simulink model "CCI"  (R2015a)
settings: Solver=ode45  StartTime=0.0  StopTime=Inf  RelTol=1e-3
libraries: commfilt2 x6, commdigbbndam3 x3, commrandsrc2 x2, commchan3 x1, commsink2 x1
settings Model: Creator=konstantis  LastModifiedBy=arlim

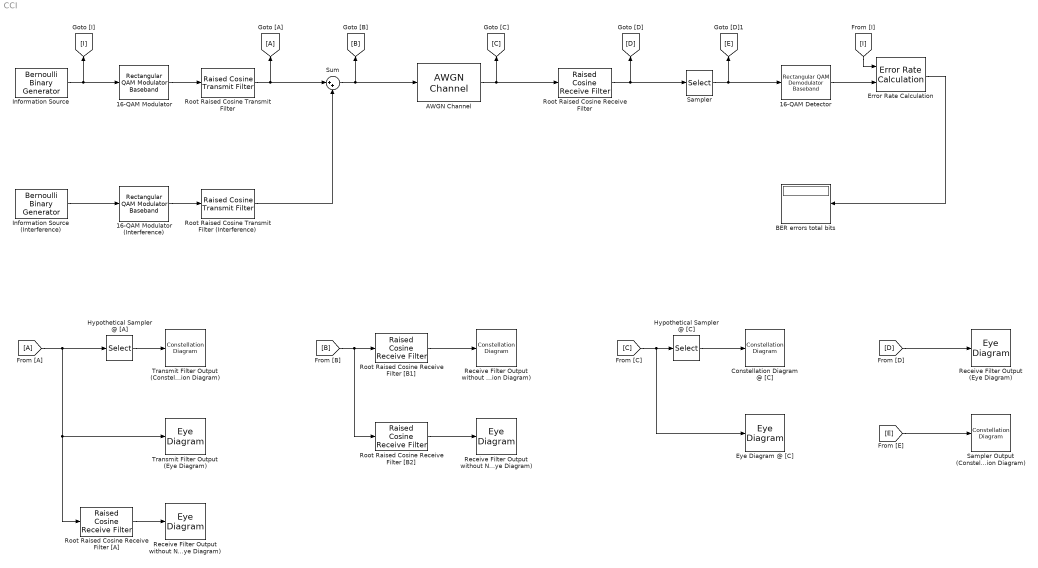
== system CCI ==
  16-QAM Detector : commdigbbndam3/Rectangular QAM Demodulator Baseband  M=16  PowType=Average Power  MinDist=2  AvgPow=1  PeakPow=1  Ph=0  Dec=Gray  Mapping=[0:15]  OutType=Bit  DecType=Hard decision  VarSource=Dialog  Variance=1  outDtype1=Inherit via internal rule  outDtype2=Inherit via internal rule  derotateFactorWordLen=16  denormFactorWordLen=16  prodOutWordLen=32  prodOutRoundingMode=Floor  prodOutOverflowMode=Wrap  sumWordLen=32
  16-QAM Modulator : commdigbbndam3/Rectangular QAM Modulator Baseband  M=16  InType=Bit  Enc=Gray  Mapping=[0:15]  PowType=Average Power  MinDist=2  AvgPow=1  PeakPow=1  Ph=0  outDtype=double  outWordLen=16  outUDDataType=sfix(16)  outFracLenMode=Best precision  outFracLen=15
  16-QAM Modulator (Interference) : commdigbbndam3/Rectangular QAM Modulator Baseband  M=16  InType=Bit  Enc=Gray  Mapping=[0:15]  PowType=Average Power  MinDist=2  AvgPow=.01  PeakPow=1  Ph=0  outDtype=double  outWordLen=16  outUDDataType=sfix(16)  outFracLenMode=Best precision  outFracLen=15
  AWGN Channel : commchan3/AWGN Channel  InputProcessing=Columns as channels (frame based)  seed=67  noiseMode="Signal to noise ratio  (SNR)"  EbNodB=10  EsNodB=10  SNRdB=15  bitsPerSym=1  Ps=1.01  Tsym=1  variance=1
  BER errors total bits : Display
      settings: Format=short_e
  Constellation Diagram @ [C] : ConstellationDiagram
  Error Rate Calculation : commsink2/Error Rate Calculation  N=128  st_delay=0  cp_mode=Entire frame  subframe=[64:10000]  PMode=Port  WsName=ErrorVec  RsMode2=off  stop=off  numErr=100  maxBits=1e6
  Eye Diagram @ [C] : EyeDiagram
  Hypothetical Sampler @ [A] : Selector  InputPortWidth=40512  Indices=[257:16:40512]
  Hypothetical Sampler @ [C] : Selector  InputPortWidth=40512  Indices=[257:16:40512]
  Information Source : commrandsrc2/Bernoulli Binary Generator  P=0.5  seed=61  Ts=1  frameBased=on  sampPerFrame=10128  orient=off  outDataType=double
  Information Source (Interference) : commrandsrc2/Bernoulli Binary Generator  P=0.5  seed=2^30  Ts=1  frameBased=on  sampPerFrame=10128  orient=off  outDataType=double
  Receive Filter Output (Eye Diagram) : EyeDiagram
  Receive Filter Output without Noise (Eye Diagram) : EyeDiagram
  Receive Filter Output without Noise + Interference (Constellation Diagram) : ConstellationDiagram
  Receive Filter Output without Noise + Interference (Eye Diagram) : EyeDiagram
  Root Raised Cosine Receive Filter : commfilt2/Raised Cosine Receive Filter  filtType=Square root  N=16  filtSpan=32  currentFiltSpan=32  D=(32)/2  R=0.35  sampMode=Mute  saveAsFlag=0  rateMode=Downsampling  downFactor=1  downOffset=0  framing=Enforce single-rate processing  InputProcessing=Columns as channels (frame based)  checkGain=Normalized  filterGain=1  checkCoeff=off  variableName=rcRxFilt1  launchFVT=on  roundingMode=Floor  overflowMode=off
  Root Raised Cosine Receive Filter [A] : commfilt2/Raised Cosine Receive Filter  filtType=Square root  N=16  filtSpan=32  currentFiltSpan=32  D=(32)/2  R=0.35  sampMode=Mute  saveAsFlag=0  rateMode=Downsampling  downFactor=1  downOffset=0  framing=Enforce single-rate processing  InputProcessing=Columns as channels (frame based)  checkGain=Normalized  filterGain=1  checkCoeff=off  variableName=rcRxFilt  launchFVT=on  roundingMode=Floor  overflowMode=off
  Root Raised Cosine Receive Filter [B1] : commfilt2/Raised Cosine Receive Filter  filtType=Square root  N=16  filtSpan=32  currentFiltSpan=32  D=(32)/2  R=0.35  sampMode=Mute  saveAsFlag=0  rateMode=Downsampling  downFactor=16  downOffset=0  framing=Enforce single-rate processing  InputProcessing=Columns as channels (frame based)  checkGain=Normalized  filterGain=1  checkCoeff=off  variableName=rcRxFilt1  launchFVT=on  roundingMode=Floor  overflowMode=off
  Root Raised Cosine Receive Filter [B2] : commfilt2/Raised Cosine Receive Filter  filtType=Square root  N=16  filtSpan=32  currentFiltSpan=32  D=(32)/2  R=0.35  sampMode=Mute  saveAsFlag=0  rateMode=Downsampling  downFactor=1  downOffset=0  framing=Enforce single-rate processing  InputProcessing=Columns as channels (frame based)  checkGain=Normalized  filterGain=1  checkCoeff=off  variableName=rcRxFilt1  launchFVT=on  roundingMode=Floor  overflowMode=off
  Root Raised Cosine Transmit Filter : commfilt2/Raised Cosine Transmit Filter  filtType=Square root  filtSpan=32  currentFiltSpan=32  D=(32)/2  R=0.35  sampMode=Mute  saveAsFlag=0  N=16  framing=Enforce single-rate processing  InputProcessing=Columns as channels (frame based)  checkGain=Normalized  filterGain=1  checkCoeff=off  variableName=rcTxFilt  launchFVT=on  roundingMode=Floor  overflowMode=off
  Root Raised Cosine Transmit Filter (Interference) : commfilt2/Raised Cosine Transmit Filter  filtType=Square root  filtSpan=32  currentFiltSpan=32  D=(32)/2  R=0.35  sampMode=Mute  saveAsFlag=0  N=16  framing=Enforce single-rate processing  InputProcessing=Columns as channels (frame based)  checkGain=Normalized  filterGain=1  checkCoeff=off  variableName=rcTxFilt1  launchFVT=on  roundingMode=Floor  overflowMode=off
  Sampler : Selector  InputPortWidth=40512  Indices=[1:16:40512]
  Sampler Output (Constellation Diagram) : ConstellationDiagram
  Sum : Sum  Inputs=|++
  Transmit Filter Output (Constellation Diagram) : ConstellationDiagram
  Transmit Filter Output (Eye Diagram) : EyeDiagram
  wires:
  Information Source/1 -> 16-QAM Modulator/1, [I]
  Information Source (Interference)/1 -> 16-QAM Modulator (Interference)/1
  Error Rate Calculation/1 -> BER errors total bits/1
  Sum/1 -> AWGN Channel/1, [B]
  16-QAM Modulator (Interference)/1 -> Root Raised Cosine Transmit Filter (Interference)/1
  [A] -> Transmit Filter Output (Eye Diagram)/1, Root Raised Cosine Receive Filter [A]/1, Hypothetical Sampler @ [A]/1
  Root Raised Cosine Receive Filter [A]/1 -> Receive Filter Output without Noise (Eye Diagram)/1
  Root Raised Cosine Receive Filter [B1]/1 -> Receive Filter Output without Noise + Interference (Constellation Diagram)/1
  Root Raised Cosine Receive Filter/1 -> Sampler/1, [D]
  Root Raised Cosine Transmit Filter/1 -> Sum/1, [A]
  16-QAM Modulator/1 -> Root Raised Cosine Transmit Filter/1
  AWGN Channel/1 -> Root Raised Cosine Receive Filter/1, [C]
  Root Raised Cosine Transmit Filter (Interference)/1 -> Sum/2
  [E] -> Sampler Output (Constellation Diagram)/1
  Root Raised Cosine Receive Filter [B2]/1 -> Receive Filter Output without Noise + Interference (Eye Diagram)/1
  [B] -> Root Raised Cosine Receive Filter [B2]/1, Root Raised Cosine Receive Filter [B1]/1
  [D] -> Receive Filter Output (Eye Diagram)/1
  [I] -> Error Rate Calculation/1
  [C] -> Eye Diagram @ [C]/1, Hypothetical Sampler @ [C]/1
  Hypothetical Sampler @ [C]/1 -> Constellation Diagram @ [C]/1
  Sampler/1 -> [E], 16-QAM Detector/1
  16-QAM Detector/1 -> Error Rate Calculation/2
  Hypothetical Sampler @ [A]/1 -> Transmit Filter Output (Constellation Diagram)/1
